simulink model "Battery_charge_discharge_FSBB_DCDC_r2020_batterySelfDesigned"  (R2020a)
settings: Solver=ode23tb  StartTime=0.0  StopTime=1  MaxStep=2.2222222222222224E-7  RelTol=1e-3  EnableMultiTasking=on
undefined symbols (not defined in the file or in its folder): Ion, Lithium, sigbuilder_block
libraries: powerlib x175, dsparch4 x4, simulink x4, electricdrivelib x1, powerlib_meascontrol x1
(part 2 of 2)

== system Battery_charge_discharge_FSBB_DCDC_r2020_batterySelfDesigned/Battery and DC-DC converter/Subsystem/lithium ion cell (2-RC equivalent circuit model, isothermal)17 ==
  C1 : powerlib/Elements/Series RLC Branch  LConnTagsString=__new0  RConnTagsString=__new0  BranchType=C  Resistance=5  Inductance=1e-3  SetiL0=off  InitialCurrent=0  Capacitance=193  Setx0=off  InitialVoltage=80  Measurements=None
  RL1 : powerlib/Elements/Series RLC Branch  LConnTagsString=__new0  RConnTagsString=__new0  BranchType=R  Resistance=0.86e-3  Inductance=1e-3  SetiL0=off  InitialCurrent=0  Capacitance=1e-6  Setx0=off  InitialVoltage=0  Measurements=None
  RL2 : powerlib/Elements/Series RLC Branch  LConnTagsString=__new0  RConnTagsString=__new0  BranchType=R  Resistance=0.78e-3  Inductance=1e-3  SetiL0=off  InitialCurrent=0  Capacitance=1e-6  Setx0=off  InitialVoltage=0  Measurements=None
  RL3 : powerlib/Elements/Series RLC Branch  LConnTagsString=__new0  RConnTagsString=__new0  BranchType=R  Resistance=0.78e-3  Inductance=1e-3  SetiL0=off  InitialCurrent=0  Capacitance=1e-6  Setx0=off  InitialVoltage=0  Measurements=None
  "母线  " : powerlib/Electrical Sources/DC Voltage Source  Amplitude=3.2  Measurements=None
  + : PMIOPort  Tag=PMCPort  Side=Left
  - : PMIOPort  Tag=PMCPort  Port=2  Side=Right
  connections:
  RL3/LConn1 -- "母线  "/RConn1 -- C1/LConn1
  "母线  "/LConn1 -- -/RConn1
  RL2/RConn1 -- RL1/RConn1 -- +/RConn1
  RL2/LConn1 -- RL1/LConn1 -- RL3/RConn1 -- C1/RConn1

== system Battery_charge_discharge_FSBB_DCDC_r2020_batterySelfDesigned/Battery and DC-DC converter/Subsystem/lithium ion cell (2-RC equivalent circuit model, isothermal)18 ==
  C1 : powerlib/Elements/Series RLC Branch  LConnTagsString=__new0  RConnTagsString=__new0  BranchType=C  Resistance=5  Inductance=1e-3  SetiL0=off  InitialCurrent=0  Capacitance=193  Setx0=off  InitialVoltage=80  Measurements=None
  RL1 : powerlib/Elements/Series RLC Branch  LConnTagsString=__new0  RConnTagsString=__new0  BranchType=R  Resistance=0.86e-3  Inductance=1e-3  SetiL0=off  InitialCurrent=0  Capacitance=1e-6  Setx0=off  InitialVoltage=0  Measurements=None
  RL2 : powerlib/Elements/Series RLC Branch  LConnTagsString=__new0  RConnTagsString=__new0  BranchType=R  Resistance=0.78e-3  Inductance=1e-3  SetiL0=off  InitialCurrent=0  Capacitance=1e-6  Setx0=off  InitialVoltage=0  Measurements=None
  RL3 : powerlib/Elements/Series RLC Branch  LConnTagsString=__new0  RConnTagsString=__new0  BranchType=R  Resistance=0.78e-3  Inductance=1e-3  SetiL0=off  InitialCurrent=0  Capacitance=1e-6  Setx0=off  InitialVoltage=0  Measurements=None
  "母线  " : powerlib/Electrical Sources/DC Voltage Source  Amplitude=3.2  Measurements=None
  + : PMIOPort  Tag=PMCPort  Side=Left
  - : PMIOPort  Tag=PMCPort  Port=2  Side=Right
  connections:
  RL3/LConn1 -- "母线  "/RConn1 -- C1/LConn1
  "母线  "/LConn1 -- -/RConn1
  RL2/RConn1 -- RL1/RConn1 -- +/RConn1
  RL2/LConn1 -- RL1/LConn1 -- RL3/RConn1 -- C1/RConn1

== system Battery_charge_discharge_FSBB_DCDC_r2020_batterySelfDesigned/Battery and DC-DC converter/Subsystem/lithium ion cell (2-RC equivalent circuit model, isothermal)19 ==
  C1 : powerlib/Elements/Series RLC Branch  LConnTagsString=__new0  RConnTagsString=__new0  BranchType=C  Resistance=5  Inductance=1e-3  SetiL0=off  InitialCurrent=0  Capacitance=193  Setx0=off  InitialVoltage=80  Measurements=None
  RL1 : powerlib/Elements/Series RLC Branch  LConnTagsString=__new0  RConnTagsString=__new0  BranchType=R  Resistance=0.86e-3  Inductance=1e-3  SetiL0=off  InitialCurrent=0  Capacitance=1e-6  Setx0=off  InitialVoltage=0  Measurements=None
  RL2 : powerlib/Elements/Series RLC Branch  LConnTagsString=__new0  RConnTagsString=__new0  BranchType=R  Resistance=0.78e-3  Inductance=1e-3  SetiL0=off  InitialCurrent=0  Capacitance=1e-6  Setx0=off  InitialVoltage=0  Measurements=None
  RL3 : powerlib/Elements/Series RLC Branch  LConnTagsString=__new0  RConnTagsString=__new0  BranchType=R  Resistance=0.78e-3  Inductance=1e-3  SetiL0=off  InitialCurrent=0  Capacitance=1e-6  Setx0=off  InitialVoltage=0  Measurements=None
  "母线  " : powerlib/Electrical Sources/DC Voltage Source  Amplitude=3.2  Measurements=None
  + : PMIOPort  Tag=PMCPort  Side=Left
  - : PMIOPort  Tag=PMCPort  Port=2  Side=Right
  connections:
  RL3/LConn1 -- "母线  "/RConn1 -- C1/LConn1
  "母线  "/LConn1 -- -/RConn1
  RL2/RConn1 -- RL1/RConn1 -- +/RConn1
  RL2/LConn1 -- RL1/LConn1 -- RL3/RConn1 -- C1/RConn1

== system Battery_charge_discharge_FSBB_DCDC_r2020_batterySelfDesigned/Battery and DC-DC converter/Subsystem/lithium ion cell (2-RC equivalent circuit model, isothermal)2 ==
  C1 : powerlib/Elements/Series RLC Branch  LConnTagsString=__new0  RConnTagsString=__new0  BranchType=C  Resistance=5  Inductance=1e-3  SetiL0=off  InitialCurrent=0  Capacitance=193  Setx0=off  InitialVoltage=80  Measurements=None
  RL1 : powerlib/Elements/Series RLC Branch  LConnTagsString=__new0  RConnTagsString=__new0  BranchType=R  Resistance=0.86e-3  Inductance=1e-3  SetiL0=off  InitialCurrent=0  Capacitance=1e-6  Setx0=off  InitialVoltage=0  Measurements=None
  RL2 : powerlib/Elements/Series RLC Branch  LConnTagsString=__new0  RConnTagsString=__new0  BranchType=R  Resistance=0.78e-3  Inductance=1e-3  SetiL0=off  InitialCurrent=0  Capacitance=1e-6  Setx0=off  InitialVoltage=0  Measurements=None
  RL3 : powerlib/Elements/Series RLC Branch  LConnTagsString=__new0  RConnTagsString=__new0  BranchType=R  Resistance=0.78e-3  Inductance=1e-3  SetiL0=off  InitialCurrent=0  Capacitance=1e-6  Setx0=off  InitialVoltage=0  Measurements=None
  "母线  " : powerlib/Electrical Sources/DC Voltage Source  Amplitude=3.2  Measurements=None
  + : PMIOPort  Tag=PMCPort  Side=Left
  - : PMIOPort  Tag=PMCPort  Port=2  Side=Right
  connections:
  RL3/LConn1 -- "母线  "/RConn1 -- C1/LConn1
  "母线  "/LConn1 -- -/RConn1
  RL2/RConn1 -- RL1/RConn1 -- +/RConn1
  RL2/LConn1 -- RL1/LConn1 -- RL3/RConn1 -- C1/RConn1

== system Battery_charge_discharge_FSBB_DCDC_r2020_batterySelfDesigned/Battery and DC-DC converter/Subsystem/lithium ion cell (2-RC equivalent circuit model, isothermal)20 ==
  C1 : powerlib/Elements/Series RLC Branch  LConnTagsString=__new0  RConnTagsString=__new0  BranchType=C  Resistance=5  Inductance=1e-3  SetiL0=off  InitialCurrent=0  Capacitance=193  Setx0=off  InitialVoltage=80  Measurements=None
  RL1 : powerlib/Elements/Series RLC Branch  LConnTagsString=__new0  RConnTagsString=__new0  BranchType=R  Resistance=0.86e-3  Inductance=1e-3  SetiL0=off  InitialCurrent=0  Capacitance=1e-6  Setx0=off  InitialVoltage=0  Measurements=None
  RL2 : powerlib/Elements/Series RLC Branch  LConnTagsString=__new0  RConnTagsString=__new0  BranchType=R  Resistance=0.78e-3  Inductance=1e-3  SetiL0=off  InitialCurrent=0  Capacitance=1e-6  Setx0=off  InitialVoltage=0  Measurements=None
  RL3 : powerlib/Elements/Series RLC Branch  LConnTagsString=__new0  RConnTagsString=__new0  BranchType=R  Resistance=0.78e-3  Inductance=1e-3  SetiL0=off  InitialCurrent=0  Capacitance=1e-6  Setx0=off  InitialVoltage=0  Measurements=None
  "母线  " : powerlib/Electrical Sources/DC Voltage Source  Amplitude=3.2  Measurements=None
  + : PMIOPort  Tag=PMCPort  Side=Left
  - : PMIOPort  Tag=PMCPort  Port=2  Side=Right
  connections:
  RL3/LConn1 -- "母线  "/RConn1 -- C1/LConn1
  "母线  "/LConn1 -- -/RConn1
  RL2/RConn1 -- RL1/RConn1 -- +/RConn1
  RL2/LConn1 -- RL1/LConn1 -- RL3/RConn1 -- C1/RConn1

== system Battery_charge_discharge_FSBB_DCDC_r2020_batterySelfDesigned/Battery and DC-DC converter/Subsystem/lithium ion cell (2-RC equivalent circuit model, isothermal)21 ==
  C1 : powerlib/Elements/Series RLC Branch  LConnTagsString=__new0  RConnTagsString=__new0  BranchType=C  Resistance=5  Inductance=1e-3  SetiL0=off  InitialCurrent=0  Capacitance=193  Setx0=off  InitialVoltage=80  Measurements=None
  RL1 : powerlib/Elements/Series RLC Branch  LConnTagsString=__new0  RConnTagsString=__new0  BranchType=R  Resistance=0.86e-3  Inductance=1e-3  SetiL0=off  InitialCurrent=0  Capacitance=1e-6  Setx0=off  InitialVoltage=0  Measurements=None
  RL2 : powerlib/Elements/Series RLC Branch  LConnTagsString=__new0  RConnTagsString=__new0  BranchType=R  Resistance=0.78e-3  Inductance=1e-3  SetiL0=off  InitialCurrent=0  Capacitance=1e-6  Setx0=off  InitialVoltage=0  Measurements=None
  RL3 : powerlib/Elements/Series RLC Branch  LConnTagsString=__new0  RConnTagsString=__new0  BranchType=R  Resistance=0.78e-3  Inductance=1e-3  SetiL0=off  InitialCurrent=0  Capacitance=1e-6  Setx0=off  InitialVoltage=0  Measurements=None
  "母线  " : powerlib/Electrical Sources/DC Voltage Source  Amplitude=3.2  Measurements=None
  + : PMIOPort  Tag=PMCPort  Side=Left
  - : PMIOPort  Tag=PMCPort  Port=2  Side=Right
  connections:
  RL3/LConn1 -- "母线  "/RConn1 -- C1/LConn1
  "母线  "/LConn1 -- -/RConn1
  RL2/RConn1 -- RL1/RConn1 -- +/RConn1
  RL2/LConn1 -- RL1/LConn1 -- RL3/RConn1 -- C1/RConn1

== system Battery_charge_discharge_FSBB_DCDC_r2020_batterySelfDesigned/Battery and DC-DC converter/Subsystem/lithium ion cell (2-RC equivalent circuit model, isothermal)22 ==
  C1 : powerlib/Elements/Series RLC Branch  LConnTagsString=__new0  RConnTagsString=__new0  BranchType=C  Resistance=5  Inductance=1e-3  SetiL0=off  InitialCurrent=0  Capacitance=193  Setx0=off  InitialVoltage=80  Measurements=None
  RL1 : powerlib/Elements/Series RLC Branch  LConnTagsString=__new0  RConnTagsString=__new0  BranchType=R  Resistance=0.86e-3  Inductance=1e-3  SetiL0=off  InitialCurrent=0  Capacitance=1e-6  Setx0=off  InitialVoltage=0  Measurements=None
  RL2 : powerlib/Elements/Series RLC Branch  LConnTagsString=__new0  RConnTagsString=__new0  BranchType=R  Resistance=0.78e-3  Inductance=1e-3  SetiL0=off  InitialCurrent=0  Capacitance=1e-6  Setx0=off  InitialVoltage=0  Measurements=None
  RL3 : powerlib/Elements/Series RLC Branch  LConnTagsString=__new0  RConnTagsString=__new0  BranchType=R  Resistance=0.78e-3  Inductance=1e-3  SetiL0=off  InitialCurrent=0  Capacitance=1e-6  Setx0=off  InitialVoltage=0  Measurements=None
  "母线  " : powerlib/Electrical Sources/DC Voltage Source  Amplitude=3.2  Measurements=None
  + : PMIOPort  Tag=PMCPort  Side=Left
  - : PMIOPort  Tag=PMCPort  Port=2  Side=Right
  connections:
  RL3/LConn1 -- "母线  "/RConn1 -- C1/LConn1
  "母线  "/LConn1 -- -/RConn1
  RL2/RConn1 -- RL1/RConn1 -- +/RConn1
  RL2/LConn1 -- RL1/LConn1 -- RL3/RConn1 -- C1/RConn1

== system Battery_charge_discharge_FSBB_DCDC_r2020_batterySelfDesigned/Battery and DC-DC converter/Subsystem/lithium ion cell (2-RC equivalent circuit model, isothermal)23 ==
  C1 : powerlib/Elements/Series RLC Branch  LConnTagsString=__new0  RConnTagsString=__new0  BranchType=C  Resistance=5  Inductance=1e-3  SetiL0=off  InitialCurrent=0  Capacitance=193  Setx0=off  InitialVoltage=80  Measurements=None
  RL1 : powerlib/Elements/Series RLC Branch  LConnTagsString=__new0  RConnTagsString=__new0  BranchType=R  Resistance=0.86e-3  Inductance=1e-3  SetiL0=off  InitialCurrent=0  Capacitance=1e-6  Setx0=off  InitialVoltage=0  Measurements=None
  RL2 : powerlib/Elements/Series RLC Branch  LConnTagsString=__new0  RConnTagsString=__new0  BranchType=R  Resistance=0.78e-3  Inductance=1e-3  SetiL0=off  InitialCurrent=0  Capacitance=1e-6  Setx0=off  InitialVoltage=0  Measurements=None
  RL3 : powerlib/Elements/Series RLC Branch  LConnTagsString=__new0  RConnTagsString=__new0  BranchType=R  Resistance=0.78e-3  Inductance=1e-3  SetiL0=off  InitialCurrent=0  Capacitance=1e-6  Setx0=off  InitialVoltage=0  Measurements=None
  "母线  " : powerlib/Electrical Sources/DC Voltage Source  Amplitude=3.2  Measurements=None
  + : PMIOPort  Tag=PMCPort  Side=Left
  - : PMIOPort  Tag=PMCPort  Port=2  Side=Right
  connections:
  RL3/LConn1 -- "母线  "/RConn1 -- C1/LConn1
  "母线  "/LConn1 -- -/RConn1
  RL2/RConn1 -- RL1/RConn1 -- +/RConn1
  RL2/LConn1 -- RL1/LConn1 -- RL3/RConn1 -- C1/RConn1

== system Battery_charge_discharge_FSBB_DCDC_r2020_batterySelfDesigned/Battery and DC-DC converter/Subsystem/lithium ion cell (2-RC equivalent circuit model, isothermal)24 ==
  C1 : powerlib/Elements/Series RLC Branch  LConnTagsString=__new0  RConnTagsString=__new0  BranchType=C  Resistance=5  Inductance=1e-3  SetiL0=off  InitialCurrent=0  Capacitance=193  Setx0=off  InitialVoltage=80  Measurements=None
  RL1 : powerlib/Elements/Series RLC Branch  LConnTagsString=__new0  RConnTagsString=__new0  BranchType=R  Resistance=0.86e-3  Inductance=1e-3  SetiL0=off  InitialCurrent=0  Capacitance=1e-6  Setx0=off  InitialVoltage=0  Measurements=None
  RL2 : powerlib/Elements/Series RLC Branch  LConnTagsString=__new0  RConnTagsString=__new0  BranchType=R  Resistance=0.78e-3  Inductance=1e-3  SetiL0=off  InitialCurrent=0  Capacitance=1e-6  Setx0=off  InitialVoltage=0  Measurements=None
  RL3 : powerlib/Elements/Series RLC Branch  LConnTagsString=__new0  RConnTagsString=__new0  BranchType=R  Resistance=0.78e-3  Inductance=1e-3  SetiL0=off  InitialCurrent=0  Capacitance=1e-6  Setx0=off  InitialVoltage=0  Measurements=None
  "母线  " : powerlib/Electrical Sources/DC Voltage Source  Amplitude=3.2  Measurements=None
  + : PMIOPort  Tag=PMCPort  Side=Left
  - : PMIOPort  Tag=PMCPort  Port=2  Side=Right
  connections:
  RL3/LConn1 -- "母线  "/RConn1 -- C1/LConn1
  "母线  "/LConn1 -- -/RConn1
  RL2/RConn1 -- RL1/RConn1 -- +/RConn1
  RL2/LConn1 -- RL1/LConn1 -- RL3/RConn1 -- C1/RConn1

== system Battery_charge_discharge_FSBB_DCDC_r2020_batterySelfDesigned/Battery and DC-DC converter/Subsystem/lithium ion cell (2-RC equivalent circuit model, isothermal)25 ==
  C1 : powerlib/Elements/Series RLC Branch  LConnTagsString=__new0  RConnTagsString=__new0  BranchType=C  Resistance=5  Inductance=1e-3  SetiL0=off  InitialCurrent=0  Capacitance=193  Setx0=off  InitialVoltage=80  Measurements=None
  RL1 : powerlib/Elements/Series RLC Branch  LConnTagsString=__new0  RConnTagsString=__new0  BranchType=R  Resistance=0.86e-3  Inductance=1e-3  SetiL0=off  InitialCurrent=0  Capacitance=1e-6  Setx0=off  InitialVoltage=0  Measurements=None
  RL2 : powerlib/Elements/Series RLC Branch  LConnTagsString=__new0  RConnTagsString=__new0  BranchType=R  Resistance=0.78e-3  Inductance=1e-3  SetiL0=off  InitialCurrent=0  Capacitance=1e-6  Setx0=off  InitialVoltage=0  Measurements=None
  RL3 : powerlib/Elements/Series RLC Branch  LConnTagsString=__new0  RConnTagsString=__new0  BranchType=R  Resistance=0.78e-3  Inductance=1e-3  SetiL0=off  InitialCurrent=0  Capacitance=1e-6  Setx0=off  InitialVoltage=0  Measurements=None
  "母线  " : powerlib/Electrical Sources/DC Voltage Source  Amplitude=3.2  Measurements=None
  + : PMIOPort  Tag=PMCPort  Side=Left
  - : PMIOPort  Tag=PMCPort  Port=2  Side=Right
  connections:
  RL3/LConn1 -- "母线  "/RConn1 -- C1/LConn1
  "母线  "/LConn1 -- -/RConn1
  RL2/RConn1 -- RL1/RConn1 -- +/RConn1
  RL2/LConn1 -- RL1/LConn1 -- RL3/RConn1 -- C1/RConn1

== system Battery_charge_discharge_FSBB_DCDC_r2020_batterySelfDesigned/Battery and DC-DC converter/Subsystem/lithium ion cell (2-RC equivalent circuit model, isothermal)26 ==
  C1 : powerlib/Elements/Series RLC Branch  LConnTagsString=__new0  RConnTagsString=__new0  BranchType=C  Resistance=5  Inductance=1e-3  SetiL0=off  InitialCurrent=0  Capacitance=193  Setx0=off  InitialVoltage=80  Measurements=None
  RL1 : powerlib/Elements/Series RLC Branch  LConnTagsString=__new0  RConnTagsString=__new0  BranchType=R  Resistance=0.86e-3  Inductance=1e-3  SetiL0=off  InitialCurrent=0  Capacitance=1e-6  Setx0=off  InitialVoltage=0  Measurements=None
  RL2 : powerlib/Elements/Series RLC Branch  LConnTagsString=__new0  RConnTagsString=__new0  BranchType=R  Resistance=0.78e-3  Inductance=1e-3  SetiL0=off  InitialCurrent=0  Capacitance=1e-6  Setx0=off  InitialVoltage=0  Measurements=None
  RL3 : powerlib/Elements/Series RLC Branch  LConnTagsString=__new0  RConnTagsString=__new0  BranchType=R  Resistance=0.78e-3  Inductance=1e-3  SetiL0=off  InitialCurrent=0  Capacitance=1e-6  Setx0=off  InitialVoltage=0  Measurements=None
  "母线  " : powerlib/Electrical Sources/DC Voltage Source  Amplitude=3.2  Measurements=None
  + : PMIOPort  Tag=PMCPort  Side=Left
  - : PMIOPort  Tag=PMCPort  Port=2  Side=Right
  connections:
  RL3/LConn1 -- "母线  "/RConn1 -- C1/LConn1
  "母线  "/LConn1 -- -/RConn1
  RL2/RConn1 -- RL1/RConn1 -- +/RConn1
  RL2/LConn1 -- RL1/LConn1 -- RL3/RConn1 -- C1/RConn1

== system Battery_charge_discharge_FSBB_DCDC_r2020_batterySelfDesigned/Battery and DC-DC converter/Subsystem/lithium ion cell (2-RC equivalent circuit model, isothermal)27 ==
  C1 : powerlib/Elements/Series RLC Branch  LConnTagsString=__new0  RConnTagsString=__new0  BranchType=C  Resistance=5  Inductance=1e-3  SetiL0=off  InitialCurrent=0  Capacitance=193  Setx0=off  InitialVoltage=80  Measurements=None
  RL1 : powerlib/Elements/Series RLC Branch  LConnTagsString=__new0  RConnTagsString=__new0  BranchType=R  Resistance=0.86e-3  Inductance=1e-3  SetiL0=off  InitialCurrent=0  Capacitance=1e-6  Setx0=off  InitialVoltage=0  Measurements=None
  RL2 : powerlib/Elements/Series RLC Branch  LConnTagsString=__new0  RConnTagsString=__new0  BranchType=R  Resistance=0.78e-3  Inductance=1e-3  SetiL0=off  InitialCurrent=0  Capacitance=1e-6  Setx0=off  InitialVoltage=0  Measurements=None
  RL3 : powerlib/Elements/Series RLC Branch  LConnTagsString=__new0  RConnTagsString=__new0  BranchType=R  Resistance=0.78e-3  Inductance=1e-3  SetiL0=off  InitialCurrent=0  Capacitance=1e-6  Setx0=off  InitialVoltage=0  Measurements=None
  "母线  " : powerlib/Electrical Sources/DC Voltage Source  Amplitude=3.2  Measurements=None
  + : PMIOPort  Tag=PMCPort  Side=Left
  - : PMIOPort  Tag=PMCPort  Port=2  Side=Right
  connections:
  RL3/LConn1 -- "母线  "/RConn1 -- C1/LConn1
  "母线  "/LConn1 -- -/RConn1
  RL2/RConn1 -- RL1/RConn1 -- +/RConn1
  RL2/LConn1 -- RL1/LConn1 -- RL3/RConn1 -- C1/RConn1

== system Battery_charge_discharge_FSBB_DCDC_r2020_batterySelfDesigned/Battery and DC-DC converter/Subsystem/lithium ion cell (2-RC equivalent circuit model, isothermal)28 ==
  C1 : powerlib/Elements/Series RLC Branch  LConnTagsString=__new0  RConnTagsString=__new0  BranchType=C  Resistance=5  Inductance=1e-3  SetiL0=off  InitialCurrent=0  Capacitance=193  Setx0=off  InitialVoltage=80  Measurements=None
  RL1 : powerlib/Elements/Series RLC Branch  LConnTagsString=__new0  RConnTagsString=__new0  BranchType=R  Resistance=0.86e-3  Inductance=1e-3  SetiL0=off  InitialCurrent=0  Capacitance=1e-6  Setx0=off  InitialVoltage=0  Measurements=None
  RL2 : powerlib/Elements/Series RLC Branch  LConnTagsString=__new0  RConnTagsString=__new0  BranchType=R  Resistance=0.78e-3  Inductance=1e-3  SetiL0=off  InitialCurrent=0  Capacitance=1e-6  Setx0=off  InitialVoltage=0  Measurements=None
  RL3 : powerlib/Elements/Series RLC Branch  LConnTagsString=__new0  RConnTagsString=__new0  BranchType=R  Resistance=0.78e-3  Inductance=1e-3  SetiL0=off  InitialCurrent=0  Capacitance=1e-6  Setx0=off  InitialVoltage=0  Measurements=None
  "母线  " : powerlib/Electrical Sources/DC Voltage Source  Amplitude=3.2  Measurements=None
  + : PMIOPort  Tag=PMCPort  Side=Left
  - : PMIOPort  Tag=PMCPort  Port=2  Side=Right
  connections:
  RL3/LConn1 -- "母线  "/RConn1 -- C1/LConn1
  "母线  "/LConn1 -- -/RConn1
  RL2/RConn1 -- RL1/RConn1 -- +/RConn1
  RL2/LConn1 -- RL1/LConn1 -- RL3/RConn1 -- C1/RConn1

== system Battery_charge_discharge_FSBB_DCDC_r2020_batterySelfDesigned/Battery and DC-DC converter/Subsystem/lithium ion cell (2-RC equivalent circuit model, isothermal)29 ==
  C1 : powerlib/Elements/Series RLC Branch  LConnTagsString=__new0  RConnTagsString=__new0  BranchType=C  Resistance=5  Inductance=1e-3  SetiL0=off  InitialCurrent=0  Capacitance=193  Setx0=off  InitialVoltage=80  Measurements=None
  RL1 : powerlib/Elements/Series RLC Branch  LConnTagsString=__new0  RConnTagsString=__new0  BranchType=R  Resistance=0.86e-3  Inductance=1e-3  SetiL0=off  InitialCurrent=0  Capacitance=1e-6  Setx0=off  InitialVoltage=0  Measurements=None
  RL2 : powerlib/Elements/Series RLC Branch  LConnTagsString=__new0  RConnTagsString=__new0  BranchType=R  Resistance=0.78e-3  Inductance=1e-3  SetiL0=off  InitialCurrent=0  Capacitance=1e-6  Setx0=off  InitialVoltage=0  Measurements=None
  RL3 : powerlib/Elements/Series RLC Branch  LConnTagsString=__new0  RConnTagsString=__new0  BranchType=R  Resistance=0.78e-3  Inductance=1e-3  SetiL0=off  InitialCurrent=0  Capacitance=1e-6  Setx0=off  InitialVoltage=0  Measurements=None
  "母线  " : powerlib/Electrical Sources/DC Voltage Source  Amplitude=3.2  Measurements=None
  + : PMIOPort  Tag=PMCPort  Side=Left
  - : PMIOPort  Tag=PMCPort  Port=2  Side=Right
  connections:
  RL3/LConn1 -- "母线  "/RConn1 -- C1/LConn1
  "母线  "/LConn1 -- -/RConn1
  RL2/RConn1 -- RL1/RConn1 -- +/RConn1
  RL2/LConn1 -- RL1/LConn1 -- RL3/RConn1 -- C1/RConn1

== system Battery_charge_discharge_FSBB_DCDC_r2020_batterySelfDesigned/Battery and DC-DC converter/Subsystem/lithium ion cell (2-RC equivalent circuit model, isothermal)3 ==
  C1 : powerlib/Elements/Series RLC Branch  LConnTagsString=__new0  RConnTagsString=__new0  BranchType=C  Resistance=5  Inductance=1e-3  SetiL0=off  InitialCurrent=0  Capacitance=193  Setx0=off  InitialVoltage=80  Measurements=None
  RL1 : powerlib/Elements/Series RLC Branch  LConnTagsString=__new0  RConnTagsString=__new0  BranchType=R  Resistance=0.86e-3  Inductance=1e-3  SetiL0=off  InitialCurrent=0  Capacitance=1e-6  Setx0=off  InitialVoltage=0  Measurements=None
  RL2 : powerlib/Elements/Series RLC Branch  LConnTagsString=__new0  RConnTagsString=__new0  BranchType=R  Resistance=0.78e-3  Inductance=1e-3  SetiL0=off  InitialCurrent=0  Capacitance=1e-6  Setx0=off  InitialVoltage=0  Measurements=None
  RL3 : powerlib/Elements/Series RLC Branch  LConnTagsString=__new0  RConnTagsString=__new0  BranchType=R  Resistance=0.78e-3  Inductance=1e-3  SetiL0=off  InitialCurrent=0  Capacitance=1e-6  Setx0=off  InitialVoltage=0  Measurements=None
  "母线  " : powerlib/Electrical Sources/DC Voltage Source  Amplitude=3.2  Measurements=None
  + : PMIOPort  Tag=PMCPort  Side=Left
  - : PMIOPort  Tag=PMCPort  Port=2  Side=Right
  connections:
  RL3/LConn1 -- "母线  "/RConn1 -- C1/LConn1
  "母线  "/LConn1 -- -/RConn1
  RL2/RConn1 -- RL1/RConn1 -- +/RConn1
  RL2/LConn1 -- RL1/LConn1 -- RL3/RConn1 -- C1/RConn1

== system Battery_charge_discharge_FSBB_DCDC_r2020_batterySelfDesigned/Battery and DC-DC converter/Subsystem/lithium ion cell (2-RC equivalent circuit model, isothermal)30 ==
  C1 : powerlib/Elements/Series RLC Branch  LConnTagsString=__new0  RConnTagsString=__new0  BranchType=C  Resistance=5  Inductance=1e-3  SetiL0=off  InitialCurrent=0  Capacitance=193  Setx0=off  InitialVoltage=80  Measurements=None
  RL1 : powerlib/Elements/Series RLC Branch  LConnTagsString=__new0  RConnTagsString=__new0  BranchType=R  Resistance=0.86e-3  Inductance=1e-3  SetiL0=off  InitialCurrent=0  Capacitance=1e-6  Setx0=off  InitialVoltage=0  Measurements=None
  RL2 : powerlib/Elements/Series RLC Branch  LConnTagsString=__new0  RConnTagsString=__new0  BranchType=R  Resistance=0.78e-3  Inductance=1e-3  SetiL0=off  InitialCurrent=0  Capacitance=1e-6  Setx0=off  InitialVoltage=0  Measurements=None
  RL3 : powerlib/Elements/Series RLC Branch  LConnTagsString=__new0  RConnTagsString=__new0  BranchType=R  Resistance=0.78e-3  Inductance=1e-3  SetiL0=off  InitialCurrent=0  Capacitance=1e-6  Setx0=off  InitialVoltage=0  Measurements=None
  "母线  " : powerlib/Electrical Sources/DC Voltage Source  Amplitude=3.2  Measurements=None
  + : PMIOPort  Tag=PMCPort  Side=Left
  - : PMIOPort  Tag=PMCPort  Port=2  Side=Right
  connections:
  RL3/LConn1 -- "母线  "/RConn1 -- C1/LConn1
  "母线  "/LConn1 -- -/RConn1
  RL2/RConn1 -- RL1/RConn1 -- +/RConn1
  RL2/LConn1 -- RL1/LConn1 -- RL3/RConn1 -- C1/RConn1

== system Battery_charge_discharge_FSBB_DCDC_r2020_batterySelfDesigned/Battery and DC-DC converter/Subsystem/lithium ion cell (2-RC equivalent circuit model, isothermal)4 ==
  C1 : powerlib/Elements/Series RLC Branch  LConnTagsString=__new0  RConnTagsString=__new0  BranchType=C  Resistance=5  Inductance=1e-3  SetiL0=off  InitialCurrent=0  Capacitance=193  Setx0=off  InitialVoltage=80  Measurements=None
  RL1 : powerlib/Elements/Series RLC Branch  LConnTagsString=__new0  RConnTagsString=__new0  BranchType=R  Resistance=0.86e-3  Inductance=1e-3  SetiL0=off  InitialCurrent=0  Capacitance=1e-6  Setx0=off  InitialVoltage=0  Measurements=None
  RL2 : powerlib/Elements/Series RLC Branch  LConnTagsString=__new0  RConnTagsString=__new0  BranchType=R  Resistance=0.78e-3  Inductance=1e-3  SetiL0=off  InitialCurrent=0  Capacitance=1e-6  Setx0=off  InitialVoltage=0  Measurements=None
  RL3 : powerlib/Elements/Series RLC Branch  LConnTagsString=__new0  RConnTagsString=__new0  BranchType=R  Resistance=0.78e-3  Inductance=1e-3  SetiL0=off  InitialCurrent=0  Capacitance=1e-6  Setx0=off  InitialVoltage=0  Measurements=None
  "母线  " : powerlib/Electrical Sources/DC Voltage Source  Amplitude=3.2  Measurements=None
  + : PMIOPort  Tag=PMCPort  Side=Left
  - : PMIOPort  Tag=PMCPort  Port=2  Side=Right
  connections:
  RL3/LConn1 -- "母线  "/RConn1 -- C1/LConn1
  "母线  "/LConn1 -- -/RConn1
  RL2/RConn1 -- RL1/RConn1 -- +/RConn1
  RL2/LConn1 -- RL1/LConn1 -- RL3/RConn1 -- C1/RConn1

== system Battery_charge_discharge_FSBB_DCDC_r2020_batterySelfDesigned/Battery and DC-DC converter/Subsystem/lithium ion cell (2-RC equivalent circuit model, isothermal)5 ==
  C1 : powerlib/Elements/Series RLC Branch  LConnTagsString=__new0  RConnTagsString=__new0  BranchType=C  Resistance=5  Inductance=1e-3  SetiL0=off  InitialCurrent=0  Capacitance=193  Setx0=off  InitialVoltage=80  Measurements=None
  RL1 : powerlib/Elements/Series RLC Branch  LConnTagsString=__new0  RConnTagsString=__new0  BranchType=R  Resistance=0.86e-3  Inductance=1e-3  SetiL0=off  InitialCurrent=0  Capacitance=1e-6  Setx0=off  InitialVoltage=0  Measurements=None
  RL2 : powerlib/Elements/Series RLC Branch  LConnTagsString=__new0  RConnTagsString=__new0  BranchType=R  Resistance=0.78e-3  Inductance=1e-3  SetiL0=off  InitialCurrent=0  Capacitance=1e-6  Setx0=off  InitialVoltage=0  Measurements=None
  RL3 : powerlib/Elements/Series RLC Branch  LConnTagsString=__new0  RConnTagsString=__new0  BranchType=R  Resistance=0.78e-3  Inductance=1e-3  SetiL0=off  InitialCurrent=0  Capacitance=1e-6  Setx0=off  InitialVoltage=0  Measurements=None
  "母线  " : powerlib/Electrical Sources/DC Voltage Source  Amplitude=3.2  Measurements=None
  + : PMIOPort  Tag=PMCPort  Side=Left
  - : PMIOPort  Tag=PMCPort  Port=2  Side=Right
  connections:
  RL3/LConn1 -- "母线  "/RConn1 -- C1/LConn1
  "母线  "/LConn1 -- -/RConn1
  RL2/RConn1 -- RL1/RConn1 -- +/RConn1
  RL2/LConn1 -- RL1/LConn1 -- RL3/RConn1 -- C1/RConn1

== system Battery_charge_discharge_FSBB_DCDC_r2020_batterySelfDesigned/Battery and DC-DC converter/Subsystem/lithium ion cell (2-RC equivalent circuit model, isothermal)6 ==
  C1 : powerlib/Elements/Series RLC Branch  LConnTagsString=__new0  RConnTagsString=__new0  BranchType=C  Resistance=5  Inductance=1e-3  SetiL0=off  InitialCurrent=0  Capacitance=193  Setx0=off  InitialVoltage=80  Measurements=None
  RL1 : powerlib/Elements/Series RLC Branch  LConnTagsString=__new0  RConnTagsString=__new0  BranchType=R  Resistance=0.86e-3  Inductance=1e-3  SetiL0=off  InitialCurrent=0  Capacitance=1e-6  Setx0=off  InitialVoltage=0  Measurements=None
  RL2 : powerlib/Elements/Series RLC Branch  LConnTagsString=__new0  RConnTagsString=__new0  BranchType=R  Resistance=0.78e-3  Inductance=1e-3  SetiL0=off  InitialCurrent=0  Capacitance=1e-6  Setx0=off  InitialVoltage=0  Measurements=None
  RL3 : powerlib/Elements/Series RLC Branch  LConnTagsString=__new0  RConnTagsString=__new0  BranchType=R  Resistance=0.78e-3  Inductance=1e-3  SetiL0=off  InitialCurrent=0  Capacitance=1e-6  Setx0=off  InitialVoltage=0  Measurements=None
  "母线  " : powerlib/Electrical Sources/DC Voltage Source  Amplitude=3.2  Measurements=None
  + : PMIOPort  Tag=PMCPort  Side=Left
  - : PMIOPort  Tag=PMCPort  Port=2  Side=Right
  connections:
  RL3/LConn1 -- "母线  "/RConn1 -- C1/LConn1
  "母线  "/LConn1 -- -/RConn1
  RL2/RConn1 -- RL1/RConn1 -- +/RConn1
  RL2/LConn1 -- RL1/LConn1 -- RL3/RConn1 -- C1/RConn1

== system Battery_charge_discharge_FSBB_DCDC_r2020_batterySelfDesigned/Battery and DC-DC converter/Subsystem/lithium ion cell (2-RC equivalent circuit model, isothermal)7 ==
  C1 : powerlib/Elements/Series RLC Branch  LConnTagsString=__new0  RConnTagsString=__new0  BranchType=C  Resistance=5  Inductance=1e-3  SetiL0=off  InitialCurrent=0  Capacitance=193  Setx0=off  InitialVoltage=80  Measurements=None
  RL1 : powerlib/Elements/Series RLC Branch  LConnTagsString=__new0  RConnTagsString=__new0  BranchType=R  Resistance=0.86e-3  Inductance=1e-3  SetiL0=off  InitialCurrent=0  Capacitance=1e-6  Setx0=off  InitialVoltage=0  Measurements=None
  RL2 : powerlib/Elements/Series RLC Branch  LConnTagsString=__new0  RConnTagsString=__new0  BranchType=R  Resistance=0.78e-3  Inductance=1e-3  SetiL0=off  InitialCurrent=0  Capacitance=1e-6  Setx0=off  InitialVoltage=0  Measurements=None
  RL3 : powerlib/Elements/Series RLC Branch  LConnTagsString=__new0  RConnTagsString=__new0  BranchType=R  Resistance=0.78e-3  Inductance=1e-3  SetiL0=off  InitialCurrent=0  Capacitance=1e-6  Setx0=off  InitialVoltage=0  Measurements=None
  "母线  " : powerlib/Electrical Sources/DC Voltage Source  Amplitude=3.2  Measurements=None
  + : PMIOPort  Tag=PMCPort  Side=Left
  - : PMIOPort  Tag=PMCPort  Port=2  Side=Right
  connections:
  RL3/LConn1 -- "母线  "/RConn1 -- C1/LConn1
  "母线  "/LConn1 -- -/RConn1
  RL2/RConn1 -- RL1/RConn1 -- +/RConn1
  RL2/LConn1 -- RL1/LConn1 -- RL3/RConn1 -- C1/RConn1

== system Battery_charge_discharge_FSBB_DCDC_r2020_batterySelfDesigned/Battery and DC-DC converter/Subsystem/lithium ion cell (2-RC equivalent circuit model, isothermal)8 ==
  C1 : powerlib/Elements/Series RLC Branch  LConnTagsString=__new0  RConnTagsString=__new0  BranchType=C  Resistance=5  Inductance=1e-3  SetiL0=off  InitialCurrent=0  Capacitance=193  Setx0=off  InitialVoltage=80  Measurements=None
  RL1 : powerlib/Elements/Series RLC Branch  LConnTagsString=__new0  RConnTagsString=__new0  BranchType=R  Resistance=0.86e-3  Inductance=1e-3  SetiL0=off  InitialCurrent=0  Capacitance=1e-6  Setx0=off  InitialVoltage=0  Measurements=None
  RL2 : powerlib/Elements/Series RLC Branch  LConnTagsString=__new0  RConnTagsString=__new0  BranchType=R  Resistance=0.78e-3  Inductance=1e-3  SetiL0=off  InitialCurrent=0  Capacitance=1e-6  Setx0=off  InitialVoltage=0  Measurements=None
  RL3 : powerlib/Elements/Series RLC Branch  LConnTagsString=__new0  RConnTagsString=__new0  BranchType=R  Resistance=0.78e-3  Inductance=1e-3  SetiL0=off  InitialCurrent=0  Capacitance=1e-6  Setx0=off  InitialVoltage=0  Measurements=None
  "母线  " : powerlib/Electrical Sources/DC Voltage Source  Amplitude=3.2  Measurements=None
  + : PMIOPort  Tag=PMCPort  Side=Left
  - : PMIOPort  Tag=PMCPort  Port=2  Side=Right
  connections:
  RL3/LConn1 -- "母线  "/RConn1 -- C1/LConn1
  "母线  "/LConn1 -- -/RConn1
  RL2/RConn1 -- RL1/RConn1 -- +/RConn1
  RL2/LConn1 -- RL1/LConn1 -- RL3/RConn1 -- C1/RConn1

== system Battery_charge_discharge_FSBB_DCDC_r2020_batterySelfDesigned/Battery and DC-DC converter/Subsystem/lithium ion cell (2-RC equivalent circuit model, isothermal)9 ==
  C1 : powerlib/Elements/Series RLC Branch  LConnTagsString=__new0  RConnTagsString=__new0  BranchType=C  Resistance=5  Inductance=1e-3  SetiL0=off  InitialCurrent=0  Capacitance=193  Setx0=off  InitialVoltage=80  Measurements=None
  RL1 : powerlib/Elements/Series RLC Branch  LConnTagsString=__new0  RConnTagsString=__new0  BranchType=R  Resistance=0.86e-3  Inductance=1e-3  SetiL0=off  InitialCurrent=0  Capacitance=1e-6  Setx0=off  InitialVoltage=0  Measurements=None
  RL2 : powerlib/Elements/Series RLC Branch  LConnTagsString=__new0  RConnTagsString=__new0  BranchType=R  Resistance=0.78e-3  Inductance=1e-3  SetiL0=off  InitialCurrent=0  Capacitance=1e-6  Setx0=off  InitialVoltage=0  Measurements=None
  RL3 : powerlib/Elements/Series RLC Branch  LConnTagsString=__new0  RConnTagsString=__new0  BranchType=R  Resistance=0.78e-3  Inductance=1e-3  SetiL0=off  InitialCurrent=0  Capacitance=1e-6  Setx0=off  InitialVoltage=0  Measurements=None
  "母线  " : powerlib/Electrical Sources/DC Voltage Source  Amplitude=3.2  Measurements=None
  + : PMIOPort  Tag=PMCPort  Side=Left
  - : PMIOPort  Tag=PMCPort  Port=2  Side=Right
  connections:
  RL3/LConn1 -- "母线  "/RConn1 -- C1/LConn1
  "母线  "/LConn1 -- -/RConn1
  RL2/RConn1 -- RL1/RConn1 -- +/RConn1
  RL2/LConn1 -- RL1/LConn1 -- RL3/RConn1 -- C1/RConn1

== matlab function Battery_charge_discharge_FSBB_DCDC_r2020_batterySelfDesigned/Battery and DC-DC converter/MATLAB Function6 ==
  settings: updateMethod=DISCRETE
  data: i_battery_ref input; i_battery input; vc2_ref input; vc2 input; vc1 input; vin input; u1 output; iL input; io input; Ts input; u2 output
function [u1, u2] = Passivity_BC(i_battery_ref, i_battery, vc2_ref, vc2,vc1,vin,iL,io,Ts)
%% system parameters
L = 20e-6;  % Inductance 电感 20uH
C1 = 1440e-6;  % 电容大小
C2 = 1440e-6;  % 电容大小
R = vc2_ref/io;  % 负载等效电阻

zeta1 = 1;  % dumping gains
zeta2 = 0.08;

% error functions: state variable
x1 = i_battery - i_battery_ref;
x2 = vc2 - vc2_ref;

persistent iL_old vc1_old vc2_ref_old;
if isempty(iL_old)
    iL_old = 0;
    vc1_old = 0;
    vc2_ref_old = 0;

end

diL = (iL - iL_old) / Ts;
dvc1 = (vc1 - vc1_old) / Ts;
dvc2_ref = (vc2_ref - vc2_ref_old) / Ts;
%% calculate switching signal: u1,u2
u2 = 1 / iL * (iL - i_battery_ref - C1*dvc1 - x2*zeta2);
%u2 = 1 / iL * (iL - vc2/R + C2*dvc2_ref + x2*zeta2);
u1 = 1 / vin * (-L*diL + vc2_ref*(1-u2) - x1*zeta1);
iL_old = iL;
vc1_old = vc1;
vc2_ref_old = vc2_ref;

== matlab function Battery_charge_discharge_FSBB_DCDC_r2020_batterySelfDesigned/Battery and DC-DC converter/MATLAB Function7 ==
  settings: updateMethod=DISCRETE
  data: i_battery_ref input; i_battery input; vc1_ref input; vc1 input; vc2 input; vin input; u1 output; iL input; Ts input; u2 output
function [u1, u2] = Passivity_BC(i_battery_ref, i_battery, vc1_ref, vc1,vc2,vin,iL,Ts)
%% system parameters
L = 20e-6;  % Inductance 电感 20uH
C1 = 1440e-6;  % 电容大小
C2 = 1440e-6;  % 电容大小

zeta1 = 6;  % dumping gains

% error functions: state variable
x1 = i_battery - i_battery_ref;
x2 = vc1 - vc1_ref;

persistent iL_old  vc1_ref_old;
if isempty(iL_old)
    iL_old = 0;
    vc1_ref_old = 0;
end

diL = (iL - iL_old) / Ts;
dvc1_ref = (vc1_ref - vc1_ref_old) / Ts;
%% calculate switching signal: u1,u2
u2 = 1 / iL * (iL - i_battery_ref - C1*dvc1_ref - x1*zeta1);
u1 = 1 / vin * (-L*diL + vc2*(1-u2));
iL_old = iL;
vc1_ref_old = vc1_ref;

== matlab function Battery_charge_discharge_FSBB_DCDC_r2020_batterySelfDesigned/Battery and DC-DC converter/MATLAB Function1 ==
  settings: updateMethod=DISCRETE
  data: iL_ref input; u1 output; iL input; io_ref input; io input; vc input; vin input; Ts input; u2 output
function [u1, u2] = Passivity_BC(iL_ref, iL, io_ref, io,vc,vin,Ts)
%% system parameters
L = 20e-6;  % Inductance 电感 20uH
RL = 0;
Co = 1440e-6;  % 电容大小
%R = vc_ref/io;  % 负载等效电阻

zeta1 = 6;  % dumping gains
zeta2 = 6;

% error functions: state variable
x1 = iL - iL_ref;
x2 = io - io_ref;
persistent iL_ref_old vc_old;
if isempty(iL_ref_old)
    iL_ref_old = 0;
    vc_old = 0;

end

diL_ref = (iL_ref - iL_ref_old) / Ts;
dvc = (vc - vc_old) / Ts;
%% calculate switching signal: u1,u2
u2 = 1 / iL_ref * (iL_ref + dvc * Co - io_ref - x2*zeta2);
u1 = 1 / vin * (-L*diL_ref + vc*(1-u2) - x1*zeta1);
iL_ref_old = iL_ref;
vc_old = vc;

== matlab function Battery_charge_discharge_FSBB_DCDC_r2020_batterySelfDesigned/Battery and DC-DC converter/MATLAB Function ==
  settings: updateMethod=DISCRETE
  data: iL_ref input; u1 output; iL input; vc_ref input; vc input; vin input; io input; Ts input; u2 output
function [u1, u2] = Passivity_BC(iL_ref, iL, vc_ref, vc, vin, io, Ts)
%% system parameters
L = 20e-6;  % Inductance 电感 20uH
RL = 0.004;
Co = 1440e-6;  % 电容大小
R = vc_ref/io;  % 负载等效电阻

zeta1 = 6;  % dumping gains
zeta2 = 0.08; 

% error functions: state variable
x1 = iL - iL_ref;
x2 = vc - vc_ref;
persistent iL_ref_old vc_ref_old;
if isempty(iL_ref_old)
    iL_ref_old = 0;
    vc_ref_old = 0;
end

diL_ref = (iL_ref - iL_ref_old) / Ts;
dvc_ref = (vc_ref - vc_ref_old) / Ts;
%% calculate switching signal: u1,u2
u2 = 1 / iL_ref * (iL_ref - dvc_ref * Co - vc_ref/R + x2*zeta2);
u1 = 1 / vin * (L*diL_ref + RL*iL_ref + vc_ref*(1-u2) - x1*zeta1);
iL_ref_old = iL_ref;
vc_ref_old = vc_ref;

== matlab function Battery_charge_discharge_FSBB_DCDC_r2020_batterySelfDesigned/Battery and DC-DC converter/MATLAB Function2 ==
  settings: updateMethod=DISCRETE
  data: i_battery_ref input; i_battery input; iL_ref input; iL input; vc2 input; vin input; vc1 input; u1 output; Ts input; u2 output
function [u1, u2] = Passivity_BC(i_battery_ref, i_battery, iL_ref, iL,vc2,vin,vc1,Ts)
%% system parameters
L = 20e-6;  % Inductance 电感 20uH
C1 = 1440e-6;  % 电容大小
C2 = 1440e-6;  % 电容大小

zeta1 = 1.2;  % dumping gains
zeta2 = 0.2;
% error functions: state variable
x1 = i_battery - i_battery_ref;
x2 = iL - iL_ref;

persistent iL_ref_old  vc1_old;
if isempty(iL_ref_old)
    iL_ref_old = 0;
    vc1_old = 0;
end

diL_ref = (iL_ref - iL_ref_old) / Ts;
dvc1 = (vc1 - vc1_old) / Ts;
%% calculate switching signal: u1,u2
u2 = 1 / iL_ref * (iL_ref - i_battery_ref - C1*dvc1 - x2*zeta2);
u1 = 1 / vin * (-L*diL_ref + vc2*(1-u2) + x1*zeta1);
iL_ref_old = iL_ref;
vc1_old = vc1;

== matlab function Battery_charge_discharge_FSBB_DCDC_r2020_batterySelfDesigned/Battery and DC-DC converter/MATLAB Function3 ==
  settings: updateMethod=DISCRETE
  data: i_battery_ref input; i_battery input; vc2_ref input; vc2 input; vc1 input; vin input; u1 output; iL input; io input; Ts input; u2 output
function [u1, u2] = Passivity_BC(i_battery_ref, i_battery, vc2_ref, vc2,vc1,vin,iL,io,Ts)
%% system parameters
L = 20e-6;  % Inductance 电感 20uH
C1 = 1440e-6;  % 电容大小
C2 = 1440e-6;  % 电容大小
R = vc2_ref/io;  % 负载等效电阻

zeta1 = 1;  % dumping gains
zeta2 = 0.08;

% error functions: state variable
x1 = i_battery - i_battery_ref;
x2 = vc2 - vc2_ref;

persistent iL_old vc1_old vc2_ref_old;
if isempty(iL_old)
    iL_old = 0;
    vc1_old = 0;
    vc2_ref_old = 0;

end

diL = (iL - iL_old) / Ts;
dvc1 = (vc1 - vc1_old) / Ts;
dvc2_ref = (vc2_ref - vc2_ref_old) / Ts;
%% calculate switching signal: u1,u2
u2 = 1 / iL * (iL - i_battery_ref - C1*dvc1 - x2*zeta2);
%u2 = 1 / iL * (iL - vc2/R + C2*dvc2_ref + x2*zeta2);
u1 = 1 / vin * (-L*diL + vc2_ref*(1-u2) - x1*zeta1);
iL_old = iL;
vc1_old = vc1;
vc2_ref_old = vc2_ref;

== matlab function Battery_charge_discharge_FSBB_DCDC_r2020_batterySelfDesigned/Battery and DC-DC converter/MATLAB Function4 ==
  settings: updateMethod=DISCRETE
  data: i_battery_ref input; i_battery input; vc1_ref input; vc1 input; vc2 input; vin input; u1 output; iL input; Ts input; u2 output
function [u1, u2] = Passivity_BC(i_battery_ref, i_battery, vc1_ref, vc1,vc2,vin,iL,Ts)
%% system parameters
L = 20e-6;  % Inductance 电感 20uH
C1 = 1440e-6;  % 电容大小
C2 = 1440e-6;  % 电容大小

zeta1 = 6;  % dumping gains

% error functions: state variable
x1 = i_battery - i_battery_ref;
x2 = vc1 - vc1_ref;

persistent iL_old  vc1_ref_old;
if isempty(iL_old)
    iL_old = 0;
    vc1_ref_old = 0;
end

diL = (iL - iL_old) / Ts;
dvc1_ref = (vc1_ref - vc1_ref_old) / Ts;
%% calculate switching signal: u1,u2
u2 = 1 / iL * (iL - i_battery_ref - C1*dvc1_ref - x1*zeta1);
u1 = 1 / vin * (-L*diL + vc2*(1-u2));
iL_old = iL;
vc1_ref_old = vc1_ref;

== matlab function Battery_charge_discharge_FSBB_DCDC_r2020_batterySelfDesigned/Battery and DC-DC converter/MATLAB Function5 ==
  settings: updateMethod=DISCRETE
  data: iL_ref input; u1 output; iL input; io_ref input; io input; vc input; vin input; Ts input; u2 output
function [u1, u2] = Passivity_BC(iL_ref, iL, io_ref, io,vc,vin,Ts)
%% system parameters
L = 20e-6;  % Inductance 电感 20uH
RL = 0;
Co = 1440e-6;  % 电容大小
%R = vc_ref/io;  % 负载等效电阻

zeta1 = 6;  % dumping gains
zeta2 = 6;

% error functions: state variable
x1 = iL - iL_ref;
x2 = io - io_ref;
persistent iL_ref_old vc_old;
if isempty(iL_ref_old)
    iL_ref_old = 0;
    vc_old = 0;

end

diL_ref = (iL_ref - iL_ref_old) / Ts;
dvc = (vc - vc_old) / Ts;
%% calculate switching signal: u1,u2
u2 = 1 / iL_ref * (iL_ref + dvc * Co - io_ref - x2*zeta2);
u1 = 1 / vin * (-L*diL_ref + vc*(1-u2) - x1*zeta1);
iL_ref_old = iL_ref;
vc_old = vc;
